simulink model "RL_Rough_Structure5"  (R2023a)
settings: Solver=VariableStepAuto  StartTime=0.0  StopTime=inf  RelTol=1e-3
libraries: rllib x1
settings Model: Creator=JC  LastModifiedBy=justin.i.chen.ctr
settings DebuggingCC: UnconnectedInputMsg=warning  UnconnectedOutputMsg=warning  UnconnectedLineMsg=warning
settings ModelReferenceCC: EnableRefExpFcnMdlSchedulingChecks=on
settings RTWCC: DLArmComputeVersion=19.05

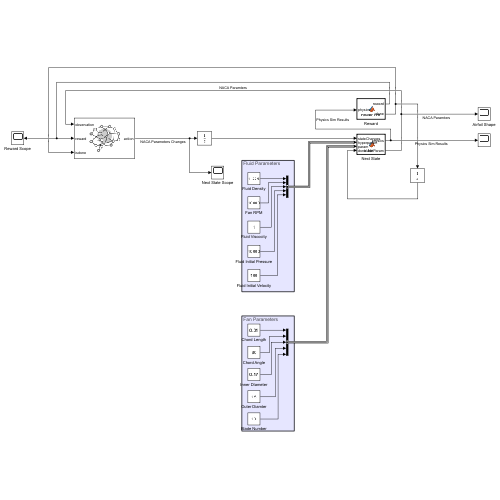
[thumbnail: Simulink's stored preview of the top-level diagram]
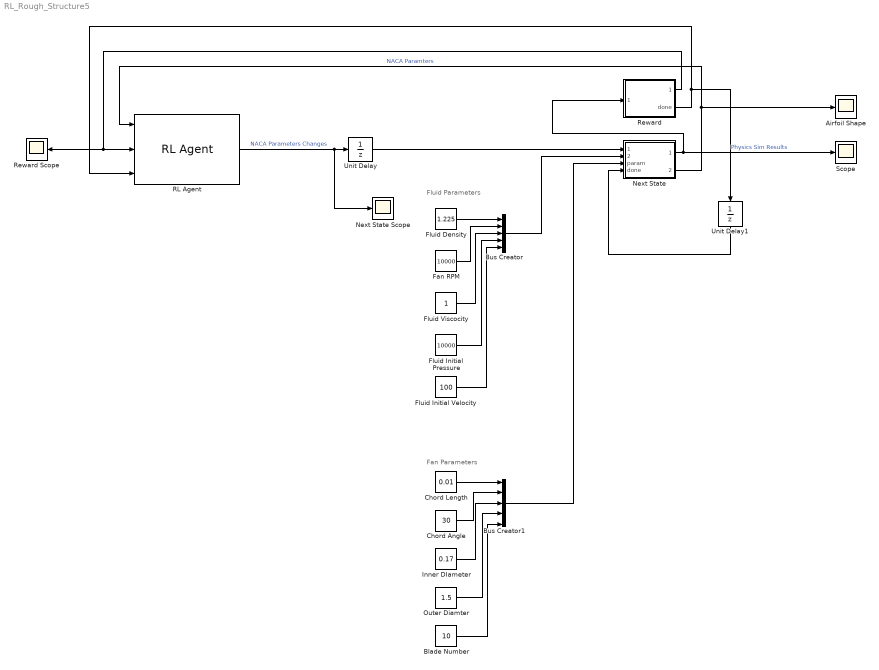
== system RL_Rough_Structure5 ==
  note: Fan Parameters
  note: Fluid Parameters
  Airfoil Shape : Scope
  Blade Number : Constant  Value=10
  Bus Creator : BusCreator  Inputs=5
  Bus Creator1 : BusCreator  Inputs=5
  Chord Angle : Constant  Value=30
  Chord Length : Constant  Value=0.01
  Fan RPM : Constant  Value=10000
  Fluid Density : Constant  Value=1.225
  Fluid Initial Pressure : Constant  Value=10000
  Fluid Initial Velocity : Constant  Value=100
  Fluid Viscocity : Constant
  Inner DIameter : Constant  Value=0.17
  Next State : MATLAB Function  TreatAsAtomicUnit=on
  Next State Scope : Scope
  Outer Diamter : Constant  Value=1.5
  RL Agent : rllib/RL Agent  Agent=agent  ExternalActionAsInput=off  ProvideLastAction=off  ProvideCumRwd=off  TreatAsDirectFeedthrough=on  UseStrictObservationDataTypes=off
  Reward : MATLAB Function  TreatAsAtomicUnit=on
  Reward Scope : Scope
  Scope : Scope
  Unit Delay : UnitDelay  SampleTime=-1  HasFrameUpgradeWarning=on
  Unit Delay1 : UnitDelay  SampleTime=-1  HasFrameUpgradeWarning=on
  wires:
  Outer Diamter/1 -> Bus Creator1/4
  Inner DIameter/1 -> Bus Creator1/3
  Blade Number/1 -> Bus Creator1/5
  Chord Angle/1 -> Bus Creator1/2
  Chord Length/1 -> Bus Creator1/1
  Fluid Density/1 -> Bus Creator/1
  Fan RPM/1 -> Bus Creator/2
  Fluid Viscocity/1 -> Bus Creator/3
  Reward/1(reward) -> Reward Scope/1, RL Agent/2
  Bus Creator1/1 -> Next State/3(param)
  Bus Creator/1 -> Next State/2(hyperparam)
  Next State/1(physics) -> Scope/1, Reward/1(physics)  "Physics Sim Results"
  Next State/2(bladeParam) -> RL Agent/1, Airfoil Shape/1  "NACA Paramters"
  RL Agent/1 -> Next State Scope/1, Unit Delay/1  "NACA Parameters Changes"
  Reward/2(done) -> Unit Delay1/1, RL Agent/3
  Fluid Initial Pressure/1 -> Bus Creator/4
  Fluid Initial Velocity/1 -> Bus Creator/5
  Unit Delay/1 -> Next State/1(stateChanges)
  Unit Delay1/1 -> Next State/4(done)

== matlab function RL_Rough_Structure5/Reward ==
  data: physics input; reward output; done output
function [reward, done] = rewardFcn(physics)
    % Extract the efficiency value from the physics input
    efficiency = physics(1);

    % Define the threshold value n
    n = 0.9;

    % Display the initial efficiency
    disp('Efficiency:');
    disp(efficiency);

    % Check if the efficiency is greater than the threshold n
    if efficiency == -1
        done = 0;
        reward = -10;
    elseif efficiency > n
        % Calculate the reward for efficiency greater than n
        reward = 10 * (efficiency - n) ^ 2;
        disp('Reward for efficiency > n:');
        disp(reward);

        % % Set the done flag to 1 (true)
        done = 1;
    else
        % Calculate the penalty for efficiency less than or equal to n
        reward = (5*efficiency - 3.5)^3;
        disp('Penalty for efficiency <= n:');
        disp(reward);

        % Set the done flag to 0 (false)
        done = 0;
    end
end
% function [reward, done] = fcn(physics)
% efficiency = physics(1);
% 
% n = 0.9;
% 
% if (efficiency > n)
%     reward = 100;
%     disp(reward);
%     done = 1;
%     return;
% elseif (efficiency > 0.5)
%     reward = 10*(efficiency-0.5);
%     disp(reward);
% else
%     reward = -((efficiency - n));%*1/n)^2 - 1;
%     disp(reward);
% end
% 
%     done = 0;
% end

== matlab function RL_Rough_Structure5/Next State ==
  data: stateChanges input; hyperparam input; physics output; bladeParam output; param input; done input
function [physics, bladeParam] = fcn(stateChanges, hyperparam, param, done)
    coder.extrinsic("fminunc");
    coder.extrinsic("optimoptions");
    coder.extrinsic("bem");
    coder.extrinsic("mxMakeArrayReal");
    coder.extrinsic("main");
    coder.extrinsic("nacaCoordinates_new");
    coder.extrinsic("xfoil");

    % nextState = size 3 array 
    % values are NACA4 parameters: 
    % all parameters in terms of chord length
    % maximum camber length (0 to 1), 
    % maximum camber position (0 to 1)
    % maximum thickness (0 to 1)

    % stateChanges = array of size 3
    % 3 naca parameter changes by agent

    % hyperparam = size 5 array of fluid parameters

    % param = size 5 array of other fan paramters

    persistent n1;
    persistent n2;
    persistent n3;
    
    if ((isempty(n1) && isempty(n2) && isempty(n3)) || done) 
        %n1 = 0.4;
        %n2 = 0.40;
        %n3 = 0.08;
        n1 = rand(1);
        n2 = rand(1);
        n3 = rand(1);
    end

    stateChanges(1) = stateChanges(1) + n1;
    stateChanges(2) = stateChanges(2) + n2;
    stateChanges(3) = stateChanges(3) + n3;

    for i = 1:3 
        if (stateChanges(i) < 0)
            stateChanges(i) = stateChanges(i) + 1;
        elseif (stateChanges(i) > 1)
            stateChanges(i) = stateChanges(i) - 1;
        end
    end

    bladeParam = stateChanges;

    physics = [NaN, NaN];
    [eff, pwr] = main(bladeParam(1), bladeParam(2), bladeParam(3), hyperparam, param);
    physics(1) = eff;
    physics(2) = pwr;

    

%     %hyperparam
%     fluidDensity = hyperparam(1);
%     fanRPM = hyperparam(2);
%     fluidViscosity = hyperparam(3);
%     initialPressure = hyperparam(4);
%     initialVelocity = hyperparam(5);
% 
%     %fan paramters
%     chordLength = param(1);
%     chordAngle = param(2);
%     id = param(3);
%     od = param(4);
%     bladeNum = param(5);
% 
% 
% %%%%% PHYSICS %%%%%%%
% 
%     coords = nacaCoordinates_new(bladeParam(1), bladeParam(2), bladeParam(3));
% 
%     X = coords(1:200,1);
%     Y = coords(1:200,2);
%     RE=6e6;
%     MACH=0;
%     alpha=0;
% 
%     [CL, CD]=xfoil(X,Y,alpha,RE,MACH);
% 
%     CLCD = [CL, CD];
% 
%     if (converge == 0)
%         eff = -1;
%         physics = [NaN, NaN];
%         physics(1) = eff;
%         return;
%     end
% 
    %%% INPUTS FOR BEMT %%%

%     chord = 0.012;
%     stations = 10;
%     element = id/2/stations;
%     BLADE = element/2:element:(id/2-element/2);
%     BETA = 15*ones(size(BLADE));
%     CHORD = chord*ones(size(BLADE));
% 
%     avionics = 10;
%     dt = 0.1;
%     mass = 1.2;
%     gravity = 9.81;
%     Aeff = 0.11;
%     dia = id;
% 
%     n = fanRPM/60;
% 
%     v = initialVelocity;
% 
%     [thrust,torque,power] = bem(CLCD, chordAngle, CHORD, BETA, BLADE, v, fanRPM, fluidDensity, bladeNum);
% 
%     thr = 4*thrust;
%     DRAG = Aeff*CD*0.5*fluidDensity*v^2;
%     dvdt = (thr-DRAG-mass*gravity)/mass;
%     v = v+dvdt*dt;
% 
%     pwr = 4*power+mass*gravity*v+DRAG*v+avionics;
% 
%     J = v/n/dia;
%     kt=thrust/(fluidDensity*n*n*dia*dia*dia*dia);
%     kq=torque/(fluidDensity*n*n*dia*dia*dia*dia*dia);
%     eff = (J/2/pi)*kt/kq;
% 
% 
%     %eff = main(bladeParam(1),bladeParam(2), bladeParam(3));
% %%%%%%% END PHYSICS %%%%%%%
% 
     % physics = [NaN, NaN];
%     physics(1) = eff;
%     physics(2) = pwr;
% 
%     %disp(eff);
end
